simulink model "Prob7"  (R2021a)
settings: Solver=VariableStepAuto  StartTime=0.0  StopTime=10.0  RelTol=1e-3
settings Model: Creator=shubham  LastModifiedBy=shubham

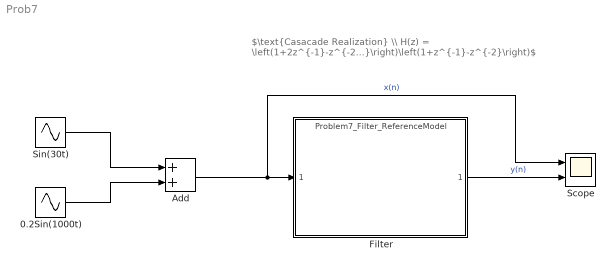
== system Prob7 ==
  note: $\text{Casacade Realization} \\ H(z) = \left(1+2z^{-1}-z^{-2}\right)\left(1+z^{-1}-z^{-2}\right)$
  0.2Sin(1000t) : Sin  Amplitude=0.2  Frequency=2*pi*1000  SampleTime=0
  Add : Sum
  Filter : ModelReference  ModelNameDialog=Problem7_Filter_ReferenceModel  SimulationMode=Normal  ModelReferenceVersion=1.5
  Scope : Scope  NumInputPorts=2
  Sin(30t) : Sin  Frequency=2*pi*30  SampleTime=0
  wires:
  0.2Sin(1000t)/1 -> Add/2
  Sin(30t)/1 -> Add/1
  Filter/1 -> Scope/2  "y(n)"
  Add/1 -> Scope/1, Filter/1  "x(n)"
